simulink model "BackStepping_ex1"  (R2021a)
settings: Solver=VariableStepAuto  StartTime=0.0  StopTime=10  RelTol=1e-3
settings Model: Creator=JianFongLee  LastModifiedBy=JianFongLee

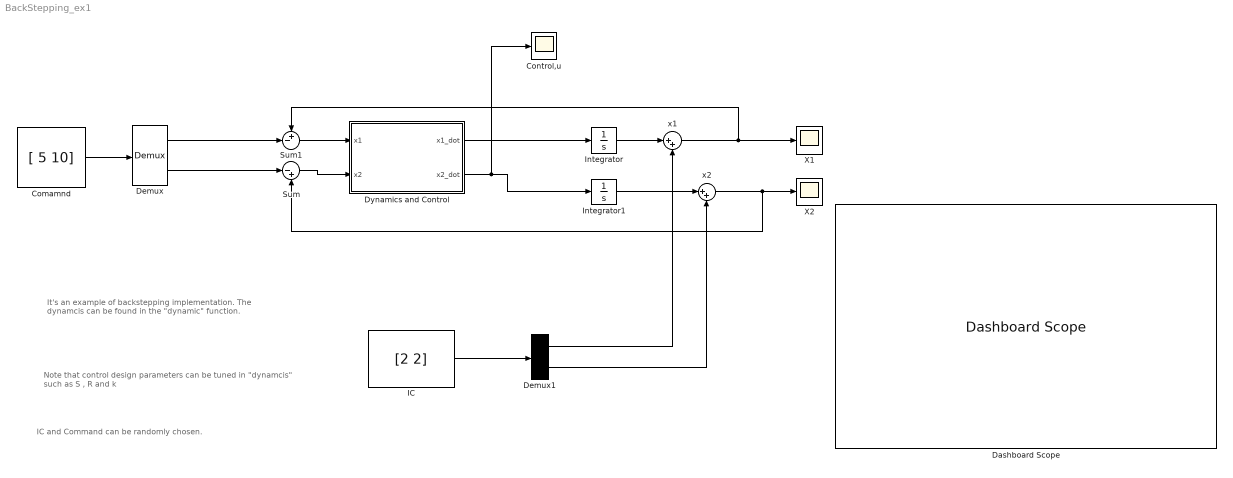
== system BackStepping_ex1 ==
  note: IC and Command can be randomly chosen.
  note: Note that control design parameters can be tuned in "dynamcis"
      | such as S , R and k
  note: It's an example of backstepping implementation.
      | The dynamcis can be found in the "dynamic" function.
  Comamnd : Constant  Value=[ 5 10]
  Control,u : Scope
  Dashboard Scope : DashboardScope
  Demux : Demux  Outputs=2
      settings: DisplayOption=none
  Demux1 : Demux  Outputs=2
      settings: DisplayOption=none
  Dynamics and Control : MATLAB Function  TreatAsAtomicUnit=on
  IC : Constant  Value=[2 2]
  Integrator : Integrator
  Integrator1 : Integrator
  Sum : Sum  Inputs=|-+
  Sum1 : Sum  Inputs=+-|
  X1 : Scope
  X2 : Scope
  x1 : Sum  Inputs=|++
  x2 : Sum  Inputs=|++
  wires:
  Comamnd/1 -> Demux/1
  Dynamics and Control/1(x1_dot) -> Integrator/1
  Dynamics and Control/2(x2_dot) -> Control,u/1, Integrator1/1
  Demux/2 -> Sum/1
  Sum/1 -> Dynamics and Control/2(x2)
  Demux/1 -> Sum1/2
  Sum1/1 -> Dynamics and Control/1(x1)
  IC/1 -> Demux1/1
  Demux1/1 -> x1/2
  Integrator/1 -> x1/1
  x1/1 -> Sum1/1, X1/1
  Integrator1/1 -> x2/1
  x2/1 -> Sum/2, X2/1
  Demux1/2 -> x2/2

== matlab function BackStepping_ex1/Dynamics and Control ==
  data: x1 input; x1_dot output; x2 input; x2_dot output
function [x1_dot,x2_dot]= dynamics(x1, x2)
%%% Parameter design here
k = 2; % Choose k > 0 
S = 1;   % S == 1 is the sweetspot
R = 5; % Maximum output of u

%%%% Control u here
P = x1 + 2*x1^3 - 2*x1^4 + 2*x1*x2;
u = -1*P - k*(x2+x1^2)^S;

%%% Add a control restriction
if abs(u) > abs(R)
   if u>0
       u = abs(R);
   else
       u = -1*abs(R);
   end
end

%%% Compute dynamics
x1_dot = x1^2 - x1^3 + x2;  % Dynamics of x1_dot
x2_dot = u;                 % Dynamics of x2_dot

%%% Lynapunov functions
%%% V1 = 0.5*x1^2 + 0.5*(x1+x2^2)^2;

%%% Notation on S, the power determines how radical V_dot is
%%% S therotically could be any odd greater than 0,
%%% but some experiments show that S = 3 or 5 would lead to oscillation
